simulink model "tapped_delay_line_customOBS"  (R2019a)
settings: Solver=ode4  StartTime=0.0  StopTime=endtime  FixedStep=0.001  RelTol=1e-3
undefined symbols (not defined in the file or in its folder): Gpd, K, L
settings Model: Creator=chris  LastModifiedBy=chris

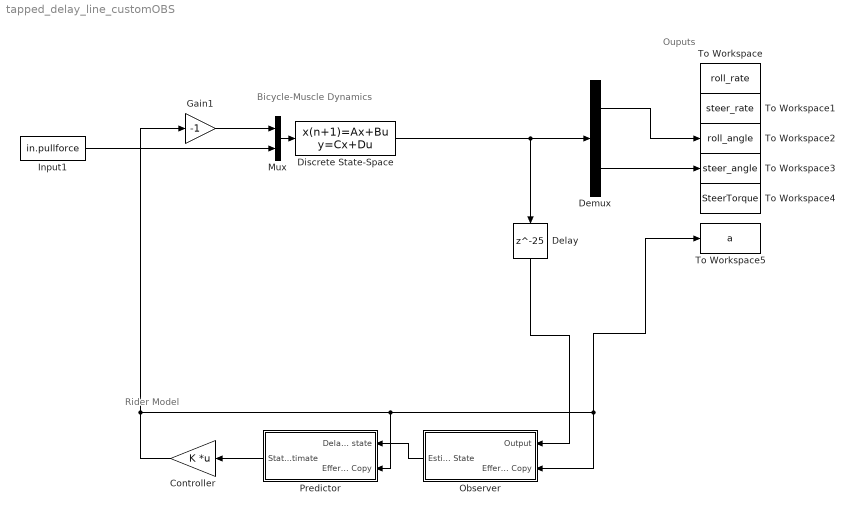
== system tapped_delay_line_customOBS ==
  note: Rider Model
  note: Ouputs
  note: Bicycle-Muscle Dynamics
  "Controller " : Gain  Gain=K  Multiplication=Matrix(K*u) (u vector)
  Delay : Delay  DelayLength=25  InitialCondition=0
  Demux : Demux  Outputs=2
  Discrete State-Space : DiscreteStateSpace  A=Gpd.A  B=Gpd.B  C=Gpd.C  D=Gpd.D  SampleTime=-1
  Gain1 : Gain  Gain=-1
  Input1 : FromWorkspace  VariableName=in.pullforce  SampleTime=0
  Mux : Mux  Inputs=2
  "Observer " : Subsystem
  "Predictor " : Subsystem
  To Workspace : ToWorkspace  VariableName=roll_rate  SampleTime=-1
  To Workspace1 : ToWorkspace  VariableName=steer_rate  SampleTime=-1
  To Workspace2 : ToWorkspace  VariableName=roll_angle  SampleTime=-1
  To Workspace3 : ToWorkspace  VariableName=steer_angle  SampleTime=-1
  To Workspace4 : ToWorkspace  VariableName=SteerTorque  SampleTime=-1
  To Workspace5 : ToWorkspace  VariableName=a  SampleTime=-1
  wires:
  Mux/1 -> Discrete State-Space/1
  Demux/2 -> To Workspace3/1
  Demux/1 -> To Workspace2/1
  Gain1/1 -> Mux/1
  Input1/1 -> Mux/2
  "Controller "/1 -> "Predictor "/2("Efference Copy "), "Observer "/2("Efference Copy "), To Workspace5/1, Gain1/1
  "Predictor "/1("State Estimate ") -> "Controller "/1
  Delay/1 -> "Observer "/1("Output ")
  Discrete State-Space/1 -> Delay/1, Demux/1
  "Observer "/1("Estimated State ") -> "Predictor "/1("Delayed state ")

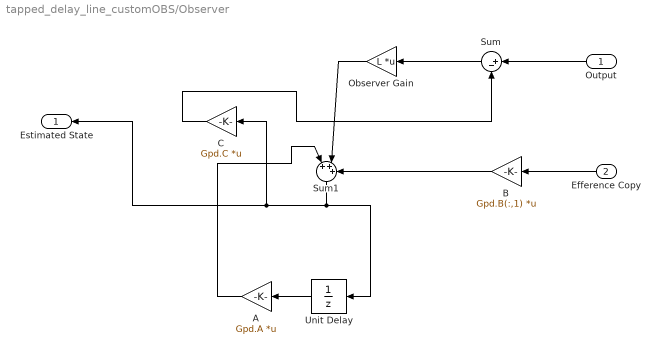
== system tapped_delay_line_customOBS/Observer  ==
  "Output " : Inport
  "Efference Copy " : Inport  Port=2
  A : Gain  Gain=Gpd.A  Multiplication=Matrix(K*u) (u vector)
  B : Gain  Gain=Gpd.B(:,1)  Multiplication=Matrix(K*u) (u vector)
  C : Gain  Gain=Gpd.C  Multiplication=Matrix(K*u) (u vector)
  "Observer Gain " : Gain  Gain=L  Multiplication=Matrix(K*u) (u vector)
  Sum : Sum  Inputs=|+-
  Sum1 : Sum  Inputs=|+++
  Unit Delay : UnitDelay  SampleTime=-1  HasFrameUpgradeWarning=on
  "Estimated State " : Outport
  wires:
  C/1 -> Sum/2
  "Output "/1 -> Sum/1
  Sum/1 -> "Observer Gain "/1
  "Efference Copy "/1 -> B/1
  B/1 -> Sum1/3
  "Observer Gain "/1 -> Sum1/2
  Sum1/1 -> Unit Delay/1, "Estimated State "/1, C/1
  A/1 -> Sum1/1
  Unit Delay/1 -> A/1

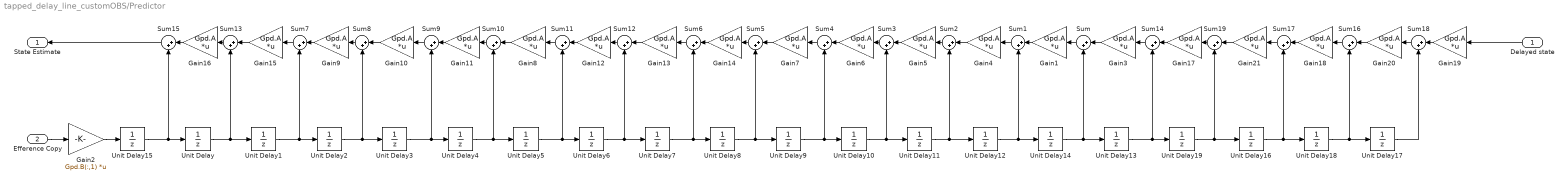
== system tapped_delay_line_customOBS/Predictor  ==
  "Delayed state " : Inport
  "Efference Copy " : Inport  Port=2
  Gain{1,3..21} (20 alike) : Gain  Gain=Gpd.A  Multiplication=Matrix(K*u) (u vector)
  Gain2 : Gain  Gain=Gpd.B(:,1)  Multiplication=Matrix(K*u) (u vector)
  Sum{,1..19} (20 alike) : Sum  Inputs=|++
  Unit Delay{,1..19} (20 alike) : UnitDelay  SampleTime=-1  HasFrameUpgradeWarning=on
  "State Estimate " : Outport
  wires:
  "Efference Copy "/1 -> Gain2/1
  Unit Delay/1 -> Sum13/2, Unit Delay1/1
  Unit Delay1/1 -> Sum7/2, Unit Delay2/1
  Unit Delay2/1 -> Sum8/2, Unit Delay3/1
  Unit Delay3/1 -> Sum9/2, Unit Delay4/1
  Unit Delay4/1 -> Sum10/2, Unit Delay5/1
  Unit Delay5/1 -> Sum11/2, Unit Delay6/1
  Unit Delay6/1 -> Sum12/2, Unit Delay7/1
  Unit Delay7/1 -> Sum6/2, Unit Delay8/1
  Unit Delay8/1 -> Sum5/2, Unit Delay9/1
  Unit Delay9/1 -> Sum4/2, Unit Delay10/1
  Unit Delay10/1 -> Sum3/2, Unit Delay11/1
  Unit Delay11/1 -> Unit Delay12/1, Sum2/2
  Unit Delay14/1 -> Unit Delay13/1, Sum/2
  Unit Delay12/1 -> Sum1/2, Unit Delay14/1
  Gain1/1 -> Sum1/1
  Sum/1 -> Gain1/1
  Gain3/1 -> Sum/1
  Sum1/1 -> Gain4/1
  Sum2/1 -> Gain5/1
  Gain4/1 -> Sum2/1
  Sum3/1 -> Gain6/1
  Gain5/1 -> Sum3/1
  Sum4/1 -> Gain7/1
  Gain6/1 -> Sum4/1
  Sum5/1 -> Gain14/1
  Gain7/1 -> Sum5/1
  Sum6/1 -> Gain13/1
  Gain14/1 -> Sum6/1
  Sum7/1 -> Gain15/1
  Gain9/1 -> Sum7/1
  Sum8/1 -> Gain9/1
  Gain10/1 -> Sum8/1
  Sum9/1 -> Gain10/1
  Gain11/1 -> Sum9/1
  Sum10/1 -> Gain11/1
  Gain8/1 -> Sum10/1
  Sum11/1 -> Gain8/1
  Gain12/1 -> Sum11/1
  Sum12/1 -> Gain12/1
  Gain13/1 -> Sum12/1
  Sum13/1 -> Gain16/1
  Gain15/1 -> Sum13/1
  Unit Delay13/1 -> Sum14/2, Unit Delay19/1
  Sum14/1 -> Gain3/1
  Gain17/1 -> Sum14/1
  Unit Delay15/1 -> Sum15/2, Unit Delay/1
  Gain2/1 -> Unit Delay15/1
  Gain16/1 -> Sum15/1
  Sum15/1 -> "State Estimate "/1
  Unit Delay18/1 -> Unit Delay17/1, Sum16/2
  Gain19/1 -> Sum18/1
  Unit Delay17/1 -> Sum18/2
  Unit Delay16/1 -> Sum17/2, Unit Delay18/1
  Gain18/1 -> Sum17/1
  Sum17/1 -> Gain21/1
  Sum16/1 -> Gain18/1
  Gain20/1 -> Sum16/1
  Sum18/1 -> Gain20/1
  "Delayed state "/1 -> Gain19/1
  Unit Delay19/1 -> Unit Delay16/1, Sum19/2
  Sum19/1 -> Gain17/1
  Gain21/1 -> Sum19/1
